simulink model "EulerPIDTunning"  (Simulink 7.6)
settings: Solver=ode3  StartTime=0.0  StopTime=2  FixedStep=Ts  RelTol=1e-3
InitFcn:
  | eval('Config');
  | eval('RobotCtlCfg');
values from neighbouring files (symbols this model uses):
  a2 = 0    [Config.m]    (also in CtrPlatformCfg.m)
  a3 = 0    [Config.m]    (also in CtrPlatformCfg.m)
  a4 = 0    [Config.m]    (also in CtrPlatformCfg.m)
  a5 = 90    [Config.m]    (also in CtrPlatformCfg.m)
  a6 = 0    [Config.m]    (also in CtrPlatformCfg.m)
  freq = tvel/radius    (= 1)    [Config.m]    (also in CtrPlatformCfg.m)
  Gravity = 9.8    [Config.m]    (also in CtrPlatformCfg.m)
  in1 = [5.2954 -0.2565 -0.6366;-0.2565 4.7000 0.2830;-0.6366 0.2829 5.8635]    [Config.m]    (also in CtrPlatformCfg.m; DynEulerTest.m; EfDynCAD.m = [0.54  -0.01 0.23)
  in2 = [5.8840 0.0072 0.0135;0.0072 6.0178 -0.1907;0.0135 -0.1907 0.3374]    [Config.m]    (also in CtrPlatformCfg.m; DynEulerTest.m; EfDynCAD.m = (R_x*R_z)*in2*(R_x*R_z)')
  in3 = [1.8201 -0.2274 -0.3112;-0.2274 2.2537 -0.1441;-0.3112 -0.1441 1.9485]    [Config.m]    (also in CtrPlatformCfg.m; DynEulerTest.m; EfDynCAD.m = (R_x*R_z)*in3*(R_x*R_z)')
  in4 = [0.0607 -0.0922 0;-0.0922 1.4493 0;0 0 1.4620]    [Config.m]    (also in CtrPlatformCfg.m; DynEulerTest.m = [0.0607 -0.0922 0;-0.0922 1.4493 0;0 0,1.4620]; EfDynCAD.m = (R_y*Rz)*in4*(R_y*Rz)')
  in5 = [0.0191 0.0032 0;0.0032 0.0228 0;0 0 0.0291]    [Config.m]    (also in CtrPlatformCfg.m; DynEulerTest.m; EfDynCAD.m = (R_x*R_y)*in5*(R_x*R_y)')
  in6 = [0.0012 0 0;0 0.0007 0;0 0 0.0007]    [Config.m]    (also in CtrPlatformCfg.m; DynEulerTest.m; EfDynCAD.m = (R_y*Rz)*in6*(R_y*Rz)')
  init_Endx = gd_init(1,4)    [Config.m]    (also in CtrPlatformCfg.m)
  init_Endy = gd_init(2,4)    [Config.m]    (also in CtrPlatformCfg.m)
  init_Endz = gd_init(3,4)    [Config.m]    (also in CtrPlatformCfg.m)
  init_Rot = gd_init(1:3,1:3)    [Config.m]    (also in CtrPlatformCfg.m)
  L = [l1 l2 l3 l4 l5 l6 l7 l8 l9]    [Config.m]    (also in CtrPlatformCfg.m)
  ma1 = 170.31    [Config.m]    (also in CtrPlatformCfg.m; DynEulerTest.m; EfDynCAD.m = 77.75)
  ma2 = 63.74    [Config.m]    (also in CtrPlatformCfg.m; DynEulerTest.m; EfDynCAD.m = 32.31)
  ma3 = 98.98    [Config.m]    (also in CtrPlatformCfg.m; DynEulerTest.m; EfDynCAD.m = 18.61)
  ma4 = 24.46    [Config.m]    (also in CtrPlatformCfg.m; DynEulerTest.m; EfDynCAD.m = 15.65)
  ma5 = 5.24    [Config.m]    (also in CtrPlatformCfg.m; DynEulerTest.m; EfDynCAD.m = 3.32)
  ma6 = 0.6    [Config.m]    (also in CtrPlatformCfg.m; DynEulerTest.m; EfDynCAD.m)
  Rad2Line = Gear*EncRes/(2*pi)    [Config.m]    (also in CtrPlatformCfg.m)
  Ts = 1/FrHz    (= 0.00025)    [Config.m]    (also in CtrPlatformCfg.m)
  tvel = 120    [Config.m]    (also in CtrPlatformCfg.m)
undefined symbols (not defined in the file or in its folder): a1, DiscIntNeverNeededParam, PRBSGain, PRBSOffset, PRBSTimeLength, PulseFrq, PulseGain, RobotAxis, SineFrq, SineGain, V2T
libraries: simulink x55, mblibv1 x35, powerlib_extras x7
(part 3 of 3)

== system EulerPIDTunning/Trajectory Generator/Still/Re-group  ==
  JJVVAA : Inport
  Demux2 : Demux  Outputs=18
  Mux{,1..2,4..6} (6 alike) : Mux  Inputs=3
  Mux3 : Mux  Inputs=6
  JVAJVA : Outport
  wires:
  Demux2/18 -> Mux6/3
  Demux2/17 -> Mux5/3
  Demux2/16 -> Mux4/3
  Demux2/15 -> Mux2/3
  Demux2/14 -> Mux1/3
  Demux2/13 -> Mux/3
  Demux2/12 -> Mux6/2
  Demux2/11 -> Mux5/2
  Demux2/10 -> Mux4/2
  Demux2/9 -> Mux2/2
  Demux2/8 -> Mux1/2
  Demux2/7 -> Mux/2
  Demux2/6 -> Mux6/1
  Demux2/5 -> Mux5/1
  Demux2/4 -> Mux4/1
  Demux2/3 -> Mux2/1
  Demux2/2 -> Mux1/1
  Demux2/1 -> Mux/1
  Mux6/1 -> Mux3/6
  Mux5/1 -> Mux3/5
  Mux4/1 -> Mux3/4
  Mux2/1 -> Mux3/3
  Mux1/1 -> Mux3/2
  Mux/1 -> Mux3/1
  Mux3/1 -> JVAJVA/1
  JJVVAA/1 -> Demux2/1

== system EulerPIDTunning/Controller/PID Controller/Controller Axis 1/EncDiff2Vel ==
  Enc : Inport
  Add : Sum  Inputs=+-
  Discrete  2nd-Order Filter : powerlib_extras/Discrete  Control Blocks/Discrete  2nd-Order Filter  DialogController=POWERSYS.PowerSysDialog  SystemSampleTime=-1  FilterType=Lowpass  Fo=1000  Zeta=0.707  Ts=Ts  Initialize=off  Vac_Init=[0.8 -25 60]  Vdc_Init=-0.4  PlotResponse=off  param1=[1 5000 10]
  Integer Delay : simulink/Discrete/Integer Delay  NumDelays=1  InputProcessing=Inherited  vinit=a1/180*pi  samptime=-1
  Vel : Outport
  wires:
  Add/1 -> Discrete  2nd-Order Filter/1
  Discrete  2nd-Order Filter/1 -> Vel/1
  Enc/1 -> Integer Delay/1, Add/1
  Integer Delay/1 -> Add/2

== system EulerPIDTunning/Controller/PID Controller/Controller Axis 1/Error Check and Lock Error ==
  CurrentCheck : Inport
  VelocityCheck : Inport  Port=2
  Abs : Abs
  Abs1 : Abs
  Compare To Constant : simulink/Logic and Bit Operations/Compare To Constant  SystemSampleTime=-1  relop=<=  const=VelErrorCheckLimit  LogicOutDataTypeMode=uint8  ZeroCross=off
  Compare To Constant1 : simulink/Logic and Bit Operations/Compare To Constant  SystemSampleTime=-1  relop=<=  const=VLLimit *1.01  LogicOutDataTypeMode=uint8  ZeroCross=off
  Logical Operator : Logic  Inputs=3  AllPortsSameDT=off  OutDataTypeStr=boolean
  Unit Delay : UnitDelay  X0=1  SampleTime=Ts
  ErrorFlag : Outport
  wires:
  VelocityCheck/1 -> Abs/1
  CurrentCheck/1 -> Abs1/1
  Unit Delay/1 -> Logical Operator/3
  Abs/1 -> Compare To Constant/1
  Abs1/1 -> Compare To Constant1/1
  Compare To Constant1/1 -> Logical Operator/1
  Compare To Constant/1 -> Logical Operator/2
  Logical Operator/1 -> ErrorFlag/1, Unit Delay/1

== system EulerPIDTunning/Controller/PID Controller/Controller Axis 1/PosAdj ==
  Pos : Inport
  Abs : Abs
  Add : Sum  Inputs=+-
  Add1 : Sum  Inputs=+-
  Compare To Constant : simulink/Logic and Bit Operations/Compare To Constant  SystemSampleTime=-1  relop=>=  const=pi/2  LogicOutDataTypeMode=uint8  ZeroCross=off
  Constant : Constant  Value=2*pi  SampleTime=Ts
  Int : DiscreteTransferFcn  Numerator=[1 0]  Denominator=[1 -1]  InitialStates=a1/180*pi  SampleTime=Ts
  Integer Delay : simulink/Discrete/Integer Delay  NumDelays=1  InputProcessing=Inherited  vinit=a1/180*pi  samptime=-1
  Product : Product  RndMeth=Zero
  Product1 : Product  RndMeth=Zero
  Sign : Signum
  PosAdj : Outport
  wires:
  Add1/1 -> Int/1
  Pos/1 -> Add/1, Integer Delay/1
  Int/1 -> PosAdj/1
  Add/1 -> Abs/1, Add1/1, Sign/1
  Integer Delay/1 -> Add/2
  Compare To Constant/1 -> Product/2
  Product/1 -> Add1/2
  Abs/1 -> Compare To Constant/1
  Constant/1 -> Product1/2
  Product1/1 -> Product/1
  Sign/1 -> Product1/1

== system EulerPIDTunning/Controller/PID Controller/Controller Axis 1/controller: PID ==
  Error : Inport
  Add1 : Sum  Inputs=+++
  D : Gain  Gain=Kd
  Diff : simulink/Discrete/Difference  SystemSampleTime=-1  ICPrevInput=0.0  OutMin=[]  OutMax=[]  OutDataType=sfix(16)  OutScaling=2^-10  DoSatur=off
  I : Gain  Gain=Ki
  Int : DiscreteTransferFcn  Numerator=[1 0]  Denominator=[1 -1]  SampleTime=Ts
  Saturation : Saturate  UpperLimit=LimitSet  LowerLimit=-LimitSet  SampleTime=Ts
      settings: AttributesFormatString=%<UpperLimit>\n%<LowerLimit>
  Saturation1 : Saturate  UpperLimit=LimitSet  LowerLimit=-LimitSet  SampleTime=Ts
      settings: AttributesFormatString=%<UpperLimit>\n%<LowerLimit>
  p : Gain  Gain=Kp
  Ctl : Outport
  wires:
  Error/1 -> p/1, I/1, D/1
  p/1 -> Add1/1
  I/1 -> Int/1
  Add1/1 -> Ctl/1
  D/1 -> Diff/1
  Diff/1 -> Saturation1/1
  Int/1 -> Saturation/1
  Saturation/1 -> Add1/2
  Saturation1/1 -> Add1/3

== system EulerPIDTunning/Controller/PID Controller/Controller Axis 1/controller: PID1 ==
  Error : Inport
  Add1 : Sum  Inputs=+++
  D : Gain  Gain=Kd
  Diff : simulink/Discrete/Difference  SystemSampleTime=-1  ICPrevInput=0.0  OutMin=[]  OutMax=[]  OutDataType=sfix(16)  OutScaling=2^-10  DoSatur=off
  I : Gain  Gain=Ki
  Int : DiscreteTransferFcn  Numerator=[1 0]  Denominator=[1 -1]  SampleTime=Ts
  Saturation1 : Saturate  UpperLimit=LimitSet  LowerLimit=-LimitSet  SampleTime=Ts
      settings: AttributesFormatString=%<UpperLimit>\n%<LowerLimit>
  Saturation2 : Saturate  UpperLimit=LimitSet  LowerLimit=-LimitSet  SampleTime=Ts
      settings: AttributesFormatString=%<UpperLimit>\n%<LowerLimit>
  p : Gain  Gain=Kp
  Ctl : Outport
  wires:
  Int/1 -> Saturation2/1
  Diff/1 -> Saturation1/1
  D/1 -> Diff/1
  Add1/1 -> Ctl/1
  I/1 -> Int/1
  p/1 -> Add1/1
  Error/1 -> D/1, I/1, p/1
  Saturation2/1 -> Add1/2
  Saturation1/1 -> Add1/3

== system EulerPIDTunning/Controller/PID Controller/Controller Axis 2/EncDiff2Vel ==
  Enc : Inport
  Add : Sum  Inputs=+-
  Discrete  2nd-Order Filter : powerlib_extras/Discrete  Control Blocks/Discrete  2nd-Order Filter  DialogController=POWERSYS.PowerSysDialog  SystemSampleTime=-1  FilterType=Lowpass  Fo=1000  Zeta=0.707  Ts=Ts  Initialize=off  Vac_Init=[0.8 -25 60]  Vdc_Init=-0.4  PlotResponse=off  param1=[1 5000 10]
  Integer Delay : simulink/Discrete/Integer Delay  NumDelays=1  InputProcessing=Inherited  vinit=a2/180*pi  samptime=-1
  Vel : Outport
  wires:
  Integer Delay/1 -> Add/2
  Enc/1 -> Add/1, Integer Delay/1
  Discrete  2nd-Order Filter/1 -> Vel/1
  Add/1 -> Discrete  2nd-Order Filter/1

== system EulerPIDTunning/Controller/PID Controller/Controller Axis 2/Error Check and Lock Error ==
  CurrentCheck : Inport
  VelocityCheck : Inport  Port=2
  Abs : Abs
  Abs1 : Abs
  Compare To Constant : simulink/Logic and Bit Operations/Compare To Constant  SystemSampleTime=-1  relop=<=  const=VelErrorCheckLimit  LogicOutDataTypeMode=uint8  ZeroCross=off
  Compare To Constant1 : simulink/Logic and Bit Operations/Compare To Constant  SystemSampleTime=-1  relop=<=  const=VLLimit *1.01  LogicOutDataTypeMode=uint8  ZeroCross=off
  Logical Operator : Logic  Inputs=3  AllPortsSameDT=off  OutDataTypeStr=boolean
  Unit Delay : UnitDelay  X0=1  SampleTime=Ts
  ErrorFlag : Outport
  wires:
  Logical Operator/1 -> Unit Delay/1, ErrorFlag/1
  Compare To Constant/1 -> Logical Operator/2
  Compare To Constant1/1 -> Logical Operator/1
  Abs1/1 -> Compare To Constant1/1
  Abs/1 -> Compare To Constant/1
  Unit Delay/1 -> Logical Operator/3
  CurrentCheck/1 -> Abs1/1
  VelocityCheck/1 -> Abs/1

== system EulerPIDTunning/Controller/PID Controller/Controller Axis 2/PosAdj ==
  Pos : Inport
  Abs : Abs
  Add : Sum  Inputs=+-
  Add1 : Sum  Inputs=+-
  Compare To Constant : simulink/Logic and Bit Operations/Compare To Constant  SystemSampleTime=-1  relop=>=  const=pi/2  LogicOutDataTypeMode=uint8  ZeroCross=off
  Constant : Constant  Value=2*pi  SampleTime=Ts
  Int : DiscreteTransferFcn  Numerator=[1 0]  Denominator=[1 -1]  InitialStates=a2/180*pi  SampleTime=Ts
  Integer Delay : simulink/Discrete/Integer Delay  NumDelays=1  InputProcessing=Inherited  vinit=a2/180*pi  samptime=-1
  Product : Product  RndMeth=Zero
  Product1 : Product  RndMeth=Zero
  Sign : Signum
  PosAdj : Outport
  wires:
  Add1/1 -> Int/1
  Pos/1 -> Add/1, Integer Delay/1
  Int/1 -> PosAdj/1
  Add/1 -> Abs/1, Add1/1, Sign/1
  Integer Delay/1 -> Add/2
  Compare To Constant/1 -> Product/2
  Product/1 -> Add1/2
  Abs/1 -> Compare To Constant/1
  Constant/1 -> Product1/2
  Product1/1 -> Product/1
  Sign/1 -> Product1/1

== system EulerPIDTunning/Controller/PID Controller/Controller Axis 2/controller: PID ==
  Error : Inport
  Add1 : Sum  Inputs=+++
  D : Gain  Gain=Kd
  Diff : simulink/Discrete/Difference  SystemSampleTime=-1  ICPrevInput=0.0  OutMin=[]  OutMax=[]  OutDataType=sfix(16)  OutScaling=2^-10  DoSatur=off
  I : Gain  Gain=Ki
  Int : DiscreteTransferFcn  Numerator=[1 0]  Denominator=[1 -1]  SampleTime=Ts
  Saturation : Saturate  UpperLimit=LimitSet  LowerLimit=-LimitSet  SampleTime=Ts
      settings: AttributesFormatString=%<UpperLimit>\n%<LowerLimit>
  Saturation1 : Saturate  UpperLimit=LimitSet  LowerLimit=-LimitSet  SampleTime=Ts
      settings: AttributesFormatString=%<UpperLimit>\n%<LowerLimit>
  p : Gain  Gain=Kp
  Ctl : Outport
  wires:
  Saturation1/1 -> Add1/3
  Saturation/1 -> Add1/2
  Int/1 -> Saturation/1
  Diff/1 -> Saturation1/1
  D/1 -> Diff/1
  Add1/1 -> Ctl/1
  I/1 -> Int/1
  p/1 -> Add1/1
  Error/1 -> D/1, I/1, p/1

== system EulerPIDTunning/Controller/PID Controller/Controller Axis 2/controller: PID1 ==
  Error : Inport
  Add1 : Sum  Inputs=+++
  D : Gain  Gain=Kd
  Diff : simulink/Discrete/Difference  SystemSampleTime=-1  ICPrevInput=0.0  OutMin=[]  OutMax=[]  OutDataType=sfix(16)  OutScaling=2^-10  DoSatur=off
  I : Gain  Gain=Ki
  Int : DiscreteTransferFcn  Numerator=[1 0]  Denominator=[1 -1]  SampleTime=Ts
  Saturation1 : Saturate  UpperLimit=LimitSet  LowerLimit=-LimitSet  SampleTime=Ts
      settings: AttributesFormatString=%<UpperLimit>\n%<LowerLimit>
  Saturation2 : Saturate  UpperLimit=LimitSet  LowerLimit=-LimitSet  SampleTime=Ts
      settings: AttributesFormatString=%<UpperLimit>\n%<LowerLimit>
  p : Gain  Gain=Kp
  Ctl : Outport
  wires:
  Saturation1/1 -> Add1/3
  Saturation2/1 -> Add1/2
  Error/1 -> p/1, I/1, D/1
  p/1 -> Add1/1
  I/1 -> Int/1
  Add1/1 -> Ctl/1
  D/1 -> Diff/1
  Diff/1 -> Saturation1/1
  Int/1 -> Saturation2/1

== system EulerPIDTunning/Controller/PID Controller/Controller Axis 3/EncDiff2Vel ==
  Enc : Inport
  Add : Sum  Inputs=+-
  Discrete  2nd-Order Filter : powerlib_extras/Discrete  Control Blocks/Discrete  2nd-Order Filter  DialogController=POWERSYS.PowerSysDialog  SystemSampleTime=-1  FilterType=Lowpass  Fo=1000  Zeta=0.707  Ts=Ts  Initialize=off  Vac_Init=[0.8 -25 60]  Vdc_Init=-0.4  PlotResponse=off  param1=[1 5000 10]
  Integer Delay : simulink/Discrete/Integer Delay  NumDelays=1  InputProcessing=Inherited  vinit=a3/180*pi  samptime=-1
  Vel : Outport
  wires:
  Add/1 -> Discrete  2nd-Order Filter/1
  Discrete  2nd-Order Filter/1 -> Vel/1
  Enc/1 -> Integer Delay/1, Add/1
  Integer Delay/1 -> Add/2

== system EulerPIDTunning/Controller/PID Controller/Controller Axis 3/Error Check and Lock Error ==
  CurrentCheck : Inport
  VelocityCheck : Inport  Port=2
  Abs : Abs
  Abs1 : Abs
  Compare To Constant : simulink/Logic and Bit Operations/Compare To Constant  SystemSampleTime=-1  relop=<=  const=VelErrorCheckLimit  LogicOutDataTypeMode=uint8  ZeroCross=off
  Compare To Constant1 : simulink/Logic and Bit Operations/Compare To Constant  SystemSampleTime=-1  relop=<=  const=VLLimit *1.01  LogicOutDataTypeMode=uint8  ZeroCross=off
  Logical Operator : Logic  Inputs=3  AllPortsSameDT=off  OutDataTypeStr=boolean
  Unit Delay : UnitDelay  X0=1  SampleTime=Ts
  ErrorFlag : Outport
  wires:
  VelocityCheck/1 -> Abs/1
  CurrentCheck/1 -> Abs1/1
  Unit Delay/1 -> Logical Operator/3
  Abs/1 -> Compare To Constant/1
  Abs1/1 -> Compare To Constant1/1
  Compare To Constant1/1 -> Logical Operator/1
  Compare To Constant/1 -> Logical Operator/2
  Logical Operator/1 -> ErrorFlag/1, Unit Delay/1

== system EulerPIDTunning/Controller/PID Controller/Controller Axis 3/PosAdj ==
  Pos : Inport
  Abs : Abs
  Add : Sum  Inputs=+-
  Add1 : Sum  Inputs=+-
  Compare To Constant : simulink/Logic and Bit Operations/Compare To Constant  SystemSampleTime=-1  relop=>=  const=pi/2  LogicOutDataTypeMode=uint8  ZeroCross=off
  Constant : Constant  Value=2*pi  SampleTime=Ts
  Int : DiscreteTransferFcn  Numerator=[1 0]  Denominator=[1 -1]  InitialStates=a3/180*pi  SampleTime=Ts
  Integer Delay : simulink/Discrete/Integer Delay  NumDelays=1  InputProcessing=Inherited  vinit=a3/180*pi  samptime=-1
  Product : Product  RndMeth=Zero
  Product1 : Product  RndMeth=Zero
  Sign : Signum
  PosAdj : Outport
  wires:
  Add1/1 -> Int/1
  Pos/1 -> Add/1, Integer Delay/1
  Int/1 -> PosAdj/1
  Add/1 -> Abs/1, Add1/1, Sign/1
  Integer Delay/1 -> Add/2
  Compare To Constant/1 -> Product/2
  Product/1 -> Add1/2
  Abs/1 -> Compare To Constant/1
  Constant/1 -> Product1/2
  Product1/1 -> Product/1
  Sign/1 -> Product1/1

== system EulerPIDTunning/Controller/PID Controller/Controller Axis 3/controller: PID ==
  Error : Inport
  Add1 : Sum  Inputs=+++
  D : Gain  Gain=Kd
  Diff : simulink/Discrete/Difference  SystemSampleTime=-1  ICPrevInput=0.0  OutMin=[]  OutMax=[]  OutDataType=sfix(16)  OutScaling=2^-10  DoSatur=off
  I : Gain  Gain=Ki
  Int : DiscreteTransferFcn  Numerator=[1 0]  Denominator=[1 -1]  SampleTime=Ts
  Saturation : Saturate  UpperLimit=LimitSet  LowerLimit=-LimitSet  SampleTime=Ts
      settings: AttributesFormatString=%<UpperLimit>\n%<LowerLimit>
  Saturation1 : Saturate  UpperLimit=LimitSet  LowerLimit=-LimitSet  SampleTime=Ts
      settings: AttributesFormatString=%<UpperLimit>\n%<LowerLimit>
  p : Gain  Gain=Kp
  Ctl : Outport
  wires:
  Error/1 -> p/1, I/1, D/1
  p/1 -> Add1/1
  I/1 -> Int/1
  Add1/1 -> Ctl/1
  D/1 -> Diff/1
  Diff/1 -> Saturation1/1
  Int/1 -> Saturation/1
  Saturation/1 -> Add1/2
  Saturation1/1 -> Add1/3

== system EulerPIDTunning/Controller/PID Controller/Controller Axis 3/controller: PID1 ==
  Error : Inport
  Add1 : Sum  Inputs=+++
  D : Gain  Gain=Kd
  Diff : simulink/Discrete/Difference  SystemSampleTime=-1  ICPrevInput=0.0  OutMin=[]  OutMax=[]  OutDataType=sfix(16)  OutScaling=2^-10  DoSatur=off
  I : Gain  Gain=Ki
  Int : DiscreteTransferFcn  Numerator=[1 0]  Denominator=[1 -1]  SampleTime=Ts
  Saturation1 : Saturate  UpperLimit=LimitSet  LowerLimit=-LimitSet  SampleTime=Ts
      settings: AttributesFormatString=%<UpperLimit>\n%<LowerLimit>
  Saturation2 : Saturate  UpperLimit=LimitSet  LowerLimit=-LimitSet  SampleTime=Ts
      settings: AttributesFormatString=%<UpperLimit>\n%<LowerLimit>
  p : Gain  Gain=Kp
  Ctl : Outport
  wires:
  Int/1 -> Saturation2/1
  Diff/1 -> Saturation1/1
  D/1 -> Diff/1
  Add1/1 -> Ctl/1
  I/1 -> Int/1
  p/1 -> Add1/1
  Error/1 -> D/1, I/1, p/1
  Saturation2/1 -> Add1/2
  Saturation1/1 -> Add1/3

== system EulerPIDTunning/Controller/PID Controller/Controller Axis 4/EncDiff2Vel ==
  Enc : Inport
  Add : Sum  Inputs=+-
  Discrete  2nd-Order Filter : powerlib_extras/Discrete  Control Blocks/Discrete  2nd-Order Filter  DialogController=POWERSYS.PowerSysDialog  SystemSampleTime=-1  FilterType=Lowpass  Fo=1000  Zeta=0.707  Ts=Ts  Initialize=off  Vac_Init=[0.8 -25 60]  Vdc_Init=-0.4  PlotResponse=off  param1=[1 5000 10]
  Integer Delay : simulink/Discrete/Integer Delay  NumDelays=1  InputProcessing=Inherited  vinit=a4/180*pi  samptime=-1
  Vel : Outport
  wires:
  Integer Delay/1 -> Add/2
  Enc/1 -> Add/1, Integer Delay/1
  Discrete  2nd-Order Filter/1 -> Vel/1
  Add/1 -> Discrete  2nd-Order Filter/1

== system EulerPIDTunning/Controller/PID Controller/Controller Axis 4/Error Check and Lock Error ==
  CurrentCheck : Inport
  VelocityCheck : Inport  Port=2
  Abs : Abs
  Abs1 : Abs
  Compare To Constant : simulink/Logic and Bit Operations/Compare To Constant  SystemSampleTime=-1  relop=<=  const=VelErrorCheckLimit  LogicOutDataTypeMode=uint8  ZeroCross=off
  Compare To Constant1 : simulink/Logic and Bit Operations/Compare To Constant  SystemSampleTime=-1  relop=<=  const=VLLimit *1.01  LogicOutDataTypeMode=uint8  ZeroCross=off
  Logical Operator : Logic  Inputs=3  AllPortsSameDT=off  OutDataTypeStr=boolean
  Unit Delay : UnitDelay  X0=1  SampleTime=Ts
  ErrorFlag : Outport
  wires:
  Logical Operator/1 -> Unit Delay/1, ErrorFlag/1
  Compare To Constant/1 -> Logical Operator/2
  Compare To Constant1/1 -> Logical Operator/1
  Abs1/1 -> Compare To Constant1/1
  Abs/1 -> Compare To Constant/1
  Unit Delay/1 -> Logical Operator/3
  CurrentCheck/1 -> Abs1/1
  VelocityCheck/1 -> Abs/1

== system EulerPIDTunning/Controller/PID Controller/Controller Axis 4/PosAdj ==
  Pos : Inport
  Abs : Abs
  Add : Sum  Inputs=+-
  Add1 : Sum  Inputs=+-
  Compare To Constant : simulink/Logic and Bit Operations/Compare To Constant  SystemSampleTime=-1  relop=>=  const=pi/2  LogicOutDataTypeMode=uint8  ZeroCross=off
  Constant : Constant  Value=2*pi  SampleTime=Ts
  Int : DiscreteTransferFcn  Numerator=[1 0]  Denominator=[1 -1]  SampleTime=Ts
  Integer Delay : simulink/Discrete/Integer Delay  NumDelays=1  InputProcessing=Inherited  vinit=a4/180*pi  samptime=-1
  Product : Product  RndMeth=Zero
  Product1 : Product  RndMeth=Zero
  Sign : Signum
  PosAdj : Outport
  wires:
  Add1/1 -> Int/1
  Pos/1 -> Add/1, Integer Delay/1
  Int/1 -> PosAdj/1
  Add/1 -> Abs/1, Add1/1, Sign/1
  Integer Delay/1 -> Add/2
  Compare To Constant/1 -> Product/2
  Product/1 -> Add1/2
  Abs/1 -> Compare To Constant/1
  Constant/1 -> Product1/2
  Product1/1 -> Product/1
  Sign/1 -> Product1/1

== system EulerPIDTunning/Controller/PID Controller/Controller Axis 4/controller: PID ==
  Error : Inport
  Add1 : Sum  Inputs=+++
  D : Gain  Gain=Kd
  Diff : simulink/Discrete/Difference  SystemSampleTime=-1  ICPrevInput=0.0  OutMin=[]  OutMax=[]  OutDataType=sfix(16)  OutScaling=2^-10  DoSatur=off
  I : Gain  Gain=Ki
  Int : DiscreteTransferFcn  Numerator=[1 0]  Denominator=[1 -1]  SampleTime=Ts
  Saturation : Saturate  UpperLimit=LimitSet  LowerLimit=-LimitSet  SampleTime=Ts
      settings: AttributesFormatString=%<UpperLimit>\n%<LowerLimit>
  Saturation1 : Saturate  UpperLimit=LimitSet  LowerLimit=-LimitSet  SampleTime=Ts
      settings: AttributesFormatString=%<UpperLimit>\n%<LowerLimit>
  p : Gain  Gain=Kp
  Ctl : Outport
  wires:
  Saturation1/1 -> Add1/3
  Saturation/1 -> Add1/2
  Int/1 -> Saturation/1
  Diff/1 -> Saturation1/1
  D/1 -> Diff/1
  Add1/1 -> Ctl/1
  I/1 -> Int/1
  p/1 -> Add1/1
  Error/1 -> D/1, I/1, p/1

== system EulerPIDTunning/Controller/PID Controller/Controller Axis 4/controller: PID1 ==
  Error : Inport
  Add1 : Sum  Inputs=+++
  D : Gain  Gain=Kd
  Diff : simulink/Discrete/Difference  SystemSampleTime=-1  ICPrevInput=0.0  OutMin=[]  OutMax=[]  OutDataType=sfix(16)  OutScaling=2^-10  DoSatur=off
  I : Gain  Gain=Ki
  Int : DiscreteTransferFcn  Numerator=[1 0]  Denominator=[1 -1]  SampleTime=Ts
  Saturation1 : Saturate  UpperLimit=LimitSet  LowerLimit=-LimitSet  SampleTime=Ts
      settings: AttributesFormatString=%<UpperLimit>\n%<LowerLimit>
  Saturation2 : Saturate  UpperLimit=LimitSet  LowerLimit=-LimitSet  SampleTime=Ts
      settings: AttributesFormatString=%<UpperLimit>\n%<LowerLimit>
  p : Gain  Gain=Kp
  Ctl : Outport
  wires:
  Saturation1/1 -> Add1/3
  Saturation2/1 -> Add1/2
  Error/1 -> p/1, I/1, D/1
  p/1 -> Add1/1
  I/1 -> Int/1
  Add1/1 -> Ctl/1
  D/1 -> Diff/1
  Diff/1 -> Saturation1/1
  Int/1 -> Saturation2/1

== system EulerPIDTunning/Controller/PID Controller/Controller Axis 5/EncDiff2Vel ==
  Enc : Inport
  Add : Sum  Inputs=+-
  Discrete  2nd-Order Filter : powerlib_extras/Discrete  Control Blocks/Discrete  2nd-Order Filter  DialogController=POWERSYS.PowerSysDialog  SystemSampleTime=-1  FilterType=Lowpass  Fo=1000  Zeta=0.707  Ts=Ts  Initialize=off  Vac_Init=[0.8 -25 60]  Vdc_Init=-0.4  PlotResponse=off  param1=[1 5000 10]
  Integer Delay : simulink/Discrete/Integer Delay  NumDelays=1  InputProcessing=Inherited  vinit=a5/180*pi  samptime=-1
  Vel : Outport
  wires:
  Add/1 -> Discrete  2nd-Order Filter/1
  Discrete  2nd-Order Filter/1 -> Vel/1
  Enc/1 -> Integer Delay/1, Add/1
  Integer Delay/1 -> Add/2

== system EulerPIDTunning/Controller/PID Controller/Controller Axis 5/Error Check and Lock Error ==
  CurrentCheck : Inport
  VelocityCheck : Inport  Port=2
  Abs : Abs
  Abs1 : Abs
  Compare To Constant : simulink/Logic and Bit Operations/Compare To Constant  SystemSampleTime=-1  relop=<=  const=VelErrorCheckLimit  LogicOutDataTypeMode=uint8  ZeroCross=off
  Compare To Constant1 : simulink/Logic and Bit Operations/Compare To Constant  SystemSampleTime=-1  relop=<=  const=VLLimit *1.01  LogicOutDataTypeMode=uint8  ZeroCross=off
  Logical Operator : Logic  Inputs=3  AllPortsSameDT=off  OutDataTypeStr=boolean
  Unit Delay : UnitDelay  X0=1  SampleTime=Ts
  ErrorFlag : Outport
  wires:
  VelocityCheck/1 -> Abs/1
  CurrentCheck/1 -> Abs1/1
  Unit Delay/1 -> Logical Operator/3
  Abs/1 -> Compare To Constant/1
  Abs1/1 -> Compare To Constant1/1
  Compare To Constant1/1 -> Logical Operator/1
  Compare To Constant/1 -> Logical Operator/2
  Logical Operator/1 -> ErrorFlag/1, Unit Delay/1

== system EulerPIDTunning/Controller/PID Controller/Controller Axis 5/PosAdj ==
  Pos : Inport
  Abs : Abs
  Add : Sum  Inputs=+-
  Add1 : Sum  Inputs=+-
  Compare To Constant : simulink/Logic and Bit Operations/Compare To Constant  SystemSampleTime=-1  relop=>=  const=pi/2  LogicOutDataTypeMode=uint8  ZeroCross=off
  Constant : Constant  Value=2*pi  SampleTime=Ts
  Int : DiscreteTransferFcn  Numerator=[1 0]  Denominator=[1 -1]  InitialStates=a5/180*pi  SampleTime=Ts
  Integer Delay : simulink/Discrete/Integer Delay  NumDelays=1  InputProcessing=Inherited  vinit=a5/180*pi  samptime=Ts
  Product : Product  RndMeth=Zero
  Product1 : Product  RndMeth=Zero
  Sign : Signum
  PosAdj : Outport
  wires:
  Add1/1 -> Int/1
  Pos/1 -> Add/1, Integer Delay/1
  Int/1 -> PosAdj/1
  Add/1 -> Abs/1, Add1/1, Sign/1
  Integer Delay/1 -> Add/2
  Compare To Constant/1 -> Product/2
  Product/1 -> Add1/2
  Abs/1 -> Compare To Constant/1
  Constant/1 -> Product1/2
  Product1/1 -> Product/1
  Sign/1 -> Product1/1

== system EulerPIDTunning/Controller/PID Controller/Controller Axis 5/controller: PID ==
  Error : Inport
  Add1 : Sum  Inputs=+++
  D : Gain  Gain=Kd
  Diff : simulink/Discrete/Difference  SystemSampleTime=-1  ICPrevInput=0.0  OutMin=[]  OutMax=[]  OutDataType=sfix(16)  OutScaling=2^-10  DoSatur=off
  I : Gain  Gain=Ki
  Int : DiscreteTransferFcn  Numerator=[1 0]  Denominator=[1 -1]  SampleTime=Ts
  Saturation : Saturate  UpperLimit=LimitSet  LowerLimit=-LimitSet  SampleTime=Ts
      settings: AttributesFormatString=%<UpperLimit>\n%<LowerLimit>
  Saturation1 : Saturate  UpperLimit=LimitSet  LowerLimit=-LimitSet  SampleTime=Ts
      settings: AttributesFormatString=%<UpperLimit>\n%<LowerLimit>
  p : Gain  Gain=Kp
  Ctl : Outport
  wires:
  Error/1 -> p/1, I/1, D/1
  p/1 -> Add1/1
  I/1 -> Int/1
  Add1/1 -> Ctl/1
  D/1 -> Diff/1
  Diff/1 -> Saturation1/1
  Int/1 -> Saturation/1
  Saturation/1 -> Add1/2
  Saturation1/1 -> Add1/3

== system EulerPIDTunning/Controller/PID Controller/Controller Axis 5/controller: PID1 ==
  Error : Inport
  Add1 : Sum  Inputs=+++
  D : Gain  Gain=Kd
  Diff : simulink/Discrete/Difference  SystemSampleTime=-1  ICPrevInput=0.0  OutMin=[]  OutMax=[]  OutDataType=sfix(16)  OutScaling=2^-10  DoSatur=off
  I : Gain  Gain=Ki
  Int : DiscreteTransferFcn  Numerator=[1 0]  Denominator=[1 -1]  SampleTime=Ts
  Saturation1 : Saturate  UpperLimit=LimitSet  LowerLimit=-LimitSet  SampleTime=Ts
      settings: AttributesFormatString=%<UpperLimit>\n%<LowerLimit>
  Saturation2 : Saturate  UpperLimit=LimitSet  LowerLimit=-LimitSet  SampleTime=Ts
      settings: AttributesFormatString=%<UpperLimit>\n%<LowerLimit>
  p : Gain  Gain=Kp
  Ctl : Outport
  wires:
  Int/1 -> Saturation2/1
  Diff/1 -> Saturation1/1
  D/1 -> Diff/1
  Add1/1 -> Ctl/1
  I/1 -> Int/1
  p/1 -> Add1/1
  Error/1 -> D/1, I/1, p/1
  Saturation2/1 -> Add1/2
  Saturation1/1 -> Add1/3

== system EulerPIDTunning/Controller/PID Controller/Controller Axis 6/EncDiff2Vel ==
  Enc : Inport
  Add : Sum  Inputs=+-
  Discrete  2nd-Order Filter : powerlib_extras/Discrete  Control Blocks/Discrete  2nd-Order Filter  DialogController=POWERSYS.PowerSysDialog  SystemSampleTime=-1  FilterType=Lowpass  Fo=1000  Zeta=0.707  Ts=Ts  Initialize=off  Vac_Init=[0.8 -25 60]  Vdc_Init=-0.4  PlotResponse=off  param1=[1 5000 10]
  Integer Delay : simulink/Discrete/Integer Delay  NumDelays=1  InputProcessing=Inherited  vinit=a6/180*pi  samptime=-1
  Vel : Outport
  wires:
  Integer Delay/1 -> Add/2
  Enc/1 -> Add/1, Integer Delay/1
  Discrete  2nd-Order Filter/1 -> Vel/1
  Add/1 -> Discrete  2nd-Order Filter/1

== system EulerPIDTunning/Controller/PID Controller/Controller Axis 6/Error Check and Lock Error ==
  CurrentCheck : Inport
  VelocityCheck : Inport  Port=2
  Abs : Abs
  Abs1 : Abs
  Compare To Constant : simulink/Logic and Bit Operations/Compare To Constant  SystemSampleTime=-1  relop=<=  const=VelErrorCheckLimit  LogicOutDataTypeMode=uint8  ZeroCross=off
  Compare To Constant1 : simulink/Logic and Bit Operations/Compare To Constant  SystemSampleTime=-1  relop=<=  const=VLLimit *1.01  LogicOutDataTypeMode=uint8  ZeroCross=off
  Logical Operator : Logic  Inputs=3  AllPortsSameDT=off  OutDataTypeStr=boolean
  Unit Delay : UnitDelay  X0=1  SampleTime=Ts
  ErrorFlag : Outport
  wires:
  Logical Operator/1 -> Unit Delay/1, ErrorFlag/1
  Compare To Constant/1 -> Logical Operator/2
  Compare To Constant1/1 -> Logical Operator/1
  Abs1/1 -> Compare To Constant1/1
  Abs/1 -> Compare To Constant/1
  Unit Delay/1 -> Logical Operator/3
  CurrentCheck/1 -> Abs1/1
  VelocityCheck/1 -> Abs/1

== system EulerPIDTunning/Controller/PID Controller/Controller Axis 6/PosAdj ==
  Pos : Inport
  Abs : Abs
  Add : Sum  Inputs=+-
  Add1 : Sum  Inputs=+-
  Compare To Constant : simulink/Logic and Bit Operations/Compare To Constant  SystemSampleTime=-1  relop=>=  const=pi/2  LogicOutDataTypeMode=uint8  ZeroCross=off
  Constant : Constant  Value=2*pi  SampleTime=Ts
  Int : DiscreteTransferFcn  Numerator=[1 0]  Denominator=[1 -1]  InitialStates=a6/180*pi  SampleTime=Ts
  Integer Delay : simulink/Discrete/Integer Delay  NumDelays=1  InputProcessing=Inherited  vinit=a6/180*pi  samptime=-1
  Product : Product  RndMeth=Zero
  Product1 : Product  RndMeth=Zero
  Sign : Signum
  PosAdj : Outport
  wires:
  Add1/1 -> Int/1
  Pos/1 -> Add/1, Integer Delay/1
  Int/1 -> PosAdj/1
  Add/1 -> Abs/1, Add1/1, Sign/1
  Integer Delay/1 -> Add/2
  Compare To Constant/1 -> Product/2
  Product/1 -> Add1/2
  Abs/1 -> Compare To Constant/1
  Constant/1 -> Product1/2
  Product1/1 -> Product/1
  Sign/1 -> Product1/1

== system EulerPIDTunning/Controller/PID Controller/Controller Axis 6/controller: PID ==
  Error : Inport
  Add1 : Sum  Inputs=+++
  D : Gain  Gain=Kd
  Diff : simulink/Discrete/Difference  SystemSampleTime=-1  ICPrevInput=0.0  OutMin=[]  OutMax=[]  OutDataType=sfix(16)  OutScaling=2^-10  DoSatur=off
  I : Gain  Gain=Ki
  Int : DiscreteTransferFcn  Numerator=[1 0]  Denominator=[1 -1]  SampleTime=Ts
  Saturation : Saturate  UpperLimit=LimitSet  LowerLimit=-LimitSet  SampleTime=Ts
      settings: AttributesFormatString=%<UpperLimit>\n%<LowerLimit>
  Saturation1 : Saturate  UpperLimit=LimitSet  LowerLimit=-LimitSet  SampleTime=Ts
      settings: AttributesFormatString=%<UpperLimit>\n%<LowerLimit>
  p : Gain  Gain=Kp
  Ctl : Outport
  wires:
  Saturation1/1 -> Add1/3
  Saturation/1 -> Add1/2
  Int/1 -> Saturation/1
  Diff/1 -> Saturation1/1
  D/1 -> Diff/1
  Add1/1 -> Ctl/1
  I/1 -> Int/1
  p/1 -> Add1/1
  Error/1 -> D/1, I/1, p/1

== system EulerPIDTunning/Controller/PID Controller/Controller Axis 6/controller: PID1 ==
  Error : Inport
  Add1 : Sum  Inputs=+++
  D : Gain  Gain=Kd
  Diff : simulink/Discrete/Difference  SystemSampleTime=-1  ICPrevInput=0.0  OutMin=[]  OutMax=[]  OutDataType=sfix(16)  OutScaling=2^-10  DoSatur=off
  I : Gain  Gain=Ki
  Int : DiscreteTransferFcn  Numerator=[1 0]  Denominator=[1 -1]  SampleTime=Ts
  Saturation1 : Saturate  UpperLimit=LimitSet  LowerLimit=-LimitSet  SampleTime=Ts
      settings: AttributesFormatString=%<UpperLimit>\n%<LowerLimit>
  Saturation2 : Saturate  UpperLimit=LimitSet  LowerLimit=-LimitSet  SampleTime=Ts
      settings: AttributesFormatString=%<UpperLimit>\n%<LowerLimit>
  p : Gain  Gain=Kp
  Ctl : Outport
  wires:
  Saturation1/1 -> Add1/3
  Saturation2/1 -> Add1/2
  Error/1 -> p/1, I/1, D/1
  p/1 -> Add1/1
  I/1 -> Int/1
  Add1/1 -> Ctl/1
  D/1 -> Diff/1
  Diff/1 -> Saturation1/1
  Int/1 -> Saturation2/1

== system EulerPIDTunning/Controller/PID Controller/Source Model/EncDiff2Vel ==
  Enc : Inport
  Add : Sum  Inputs=+-
  Discrete  2nd-Order Filter : powerlib_extras/Discrete  Control Blocks/Discrete  2nd-Order Filter  DialogController=POWERSYS.PowerSysDialog  SystemSampleTime=-1  FilterType=Lowpass  Fo=1000  Zeta=0.707  Ts=Ts  Initialize=off  Vac_Init=[0.8 -25 60]  Vdc_Init=-0.4  PlotResponse=off  param1=[1 5000 10]
  Integer Delay : simulink/Discrete/Integer Delay  NumDelays=1  InputProcessing=Inherited  vinit=0.0  samptime=-1
  Vel : Outport
  wires:
  Integer Delay/1 -> Add/2
  Enc/1 -> Add/1, Integer Delay/1
  Discrete  2nd-Order Filter/1 -> Vel/1
  Add/1 -> Discrete  2nd-Order Filter/1

== system EulerPIDTunning/Controller/PID Controller/Source Model/source: PRBS ==
  Enable : EnablePort  StatesWhenEnabling=reset
  Add : Sum
  Gain1 : Gain  Gain=Ts
  Lookup Table : Lookup  InputValues=(0:TL/Ts)*Ts;  Table=[prbs_u; 0];  LookUpMeth=Interpolation-Use End Values  SampleTime=Ts
  PRBSGain : Gain  Gain=CurrentValue  SampleTime=Ts
  Ts : Constant  SampleTime=Ts
  Unit Delay : UnitDelay  SampleTime=Ts
  PRBS* : Outport  OutputWhenDisabled=reset  InitialOutput=0
  wires:
  Lookup Table/1 -> PRBSGain/1
  PRBSGain/1 -> PRBS*/1
  Add/1 -> Unit Delay/1, Gain1/1
  Ts/1 -> Add/2
  Unit Delay/1 -> Add/1
  Gain1/1 -> Lookup Table/1

== system EulerPIDTunning/Controller/PID Controller/Source Model/source: Pulse ==
  Enable : EnablePort  StatesWhenEnabling=reset
  Add : Sum
  Gain1 : Gain  Gain=Ts
  PulseGain : Gain  Gain=VelGain
  Sign : Signum
  Sine Wave : Sin  TimeSource=Use external signal  Frequency=Frq*2*pi  SampleTime=31.25e-6
  Ts : Constant  SampleTime=Ts
  Unit Delay : UnitDelay  SampleTime=Ts
  Vel1 : Scope
      settings: TimeRange=4.5  YMin=0.15  YMax=1  SaveName=ScopeData10
  Pulse : Outport  OutputWhenDisabled=reset  InitialOutput=0
  wires:
  Sine Wave/1 -> Sign/1, Vel1/1
  Sign/1 -> PulseGain/1
  PulseGain/1 -> Pulse/1
  Add/1 -> Unit Delay/1, Gain1/1
  Ts/1 -> Add/2
  Unit Delay/1 -> Add/1
  Gain1/1 -> Sine Wave/1

== system EulerPIDTunning/Controller/PID Controller/Source Model/source: SineSwp ==
  Enable : EnablePort  StatesWhenEnabling=reset
  AmpG : Subsystem
  Constant : Constant  Value=2*pi  SampleTime=Ts
  DelayCmp : Subsystem
  Product : Product  Inputs=3  RndMeth=Zero
  Product1 : Product  RndMeth=Zero
  Product2 : Product  RndMeth=Zero
  Product3 : Product  RndMeth=Zero
  Scope1 : Scope
      settings: TimeRange=0.05  SaveName=ScopeData3
  Scope4 : Scope
      settings: TimeRange=0.05  SaveName=ScopeData7
  SignalGen : Stateflow chart  TreatAsAtomicUnit=on
  Timer : Subsystem
  Trigonometric Function : Trigonometry  SampleTime=Ts
  Unit Delay1 : UnitDelay  X0=1  SampleTime=Ts
  Unit Delay2 : UnitDelay  SampleTime=Ts
  Unit Delay3 : UnitDelay  X0=1  SampleTime=Ts
  Unit Delay4 : UnitDelay  X0=0.01  SampleTime=Ts
  SineOut : Outport  OutputWhenDisabled=reset  InitialOutput=0
  wires:
  Timer/1(Time) -> Product/1, SignalGen/1(mytime)
  Constant/1 -> Product/2
  SignalGen/1(Frq) -> Product/3, Scope1/1, Unit Delay4/1
  Product/1 -> Trigonometric Function/1
  Product1/1 -> SineOut/1, Scope4/1
  Trigonometric Function/1 -> Product1/1
  AmpG/1(TrueAmp) -> Product1/2, Unit Delay2/1
  Unit Delay2/1 -> SignalGen/2(TureAmp)
  SignalGen/4(CounterOut) -> Unit Delay3/1
  Unit Delay3/1 -> SignalGen/3(CounterIn)
  SignalGen/3(PeriodFlag) -> Unit Delay1/1
  SignalGen/5(Ramp) -> AmpG/2(Ramp)
  Unit Delay1/1 -> DelayCmp/1(Signal), Product2/1
  SignalGen/2(Amp) -> Product3/1
  Product3/1 -> AmpG/1(Amp)
  DelayCmp/1(UnChange) -> Product2/2, Product3/2
  Product2/1 -> Timer/Enable
  Unit Delay4/1 -> DelayCmp/2(frq)

== system EulerPIDTunning/Controller/PID Controller/Source Model/source: Single ==
  Enable : EnablePort  StatesWhenEnabling=reset
  Add : Sum
  Gain1 : Gain  Gain=Ts
  Sine Wave : Sin  TimeSource=Use external signal  Frequency=Frq*2*pi  SampleTime=31.25e-6
  SineGain : Gain  Gain=VelGain
  Ts : Constant  SampleTime=Ts
  Unit Delay : UnitDelay  SampleTime=Ts
  Sine : Outport  OutputWhenDisabled=reset  InitialOutput=0
  wires:
  Sine Wave/1 -> SineGain/1
  SineGain/1 -> Sine/1
  Add/1 -> Unit Delay/1, Gain1/1
  Ts/1 -> Add/2
  Unit Delay/1 -> Add/1
  Gain1/1 -> Sine Wave/1

== system EulerPIDTunning/Controller/PID Controller/Source Model/source: SineSwp/AmpG ==
  Amp : Inport
  Ramp : Inport  Port=2
  Abs : Abs
  Add1 : Sum  Inputs=+-
  Add2 : Sum
  Product : Product  RndMeth=Zero
  Relational Operator : RelationalOperator  Operator=<=  OutDataTypeStr=boolean  SampleTime=Ts
  Sign : Signum
  Switch : Switch  Threshold=0.5
  Unit Delay1 : UnitDelay  SampleTime=Ts
  TrueAmp : Outport  InitialOutput=0
  wires:
  Add1/1 -> Abs/1, Sign/1
  Add2/1 -> Unit Delay1/1, TrueAmp/1
  Amp/1 -> Add1/1
  Unit Delay1/1 -> Add2/2, Add1/2
  Ramp/1 -> Relational Operator/1, Switch/1
  Abs/1 -> Relational Operator/2, Switch/3
  Relational Operator/1 -> Switch/2
  Switch/1 -> Product/1
  Sign/1 -> Product/2
  Product/1 -> Add2/1

== system EulerPIDTunning/Controller/PID Controller/Source Model/source: SineSwp/DelayCmp ==
  Signal : Inport
  frq : Inport  Port=2
  DelayCmp : Stateflow chart  TreatAsAtomicUnit=on
  Detect Change : simulink/Logic and Bit Operations/Detect Change  SystemSampleTime=-1  vinit=1
  UnChange : Outport
  wires:
  Signal/1 -> Detect Change/1
  Detect Change/1 -> DelayCmp/1(change)
  DelayCmp/1(output) -> UnChange/1
  frq/1 -> DelayCmp/2(frq)

== system EulerPIDTunning/Controller/PID Controller/Source Model/source: SineSwp/Timer ==
  Enable : EnablePort  StatesWhenEnabling=reset
  Add2 : Sum
  Ts : Constant  Value=Ts  SampleTime=Ts
  Unit Delay1 : UnitDelay  SampleTime=Ts
  Time : Outport  OutputWhenDisabled=reset  InitialOutput=0
  wires:
  Ts/1 -> Add2/2
  Unit Delay1/1 -> Add2/1
  Add2/1 -> Time/1, Unit Delay1/1

== matlab function Trajectory Generator/Still/Inverse Kinematic ==
  data: EndPos input double; init_Rot parameter double; Theta output double; L parameter double
function Theta = fcn(EndPos,init_Rot,L)
%#eml
Theta =[0;0; 0; 0; 0; 0];
gd = [init_Rot,EndPos;[0 0 0],1];
[Theta_total,num_total] = inv_kin(gd,L);
%%%%%%%%%%%Need to modify%%%%%%%%%%%%%%%
Theta = Theta_total(:,2);

== matlab function Trajectory Generator/Still/Jacobian ==
  data: Theta input double; Omega output double; EndVel input double; L parameter double
function Omega = fcn(Theta,EndVel,L)
%#eml

Omega = zeros(6,1);
V = [EndVel; 0; 0; 0];   
g = fwd_kin(L,Theta');
Jb = body_Jacobian(L,Theta');
Adg_inv = double(AdjointInv(g));
Omega = double((Jb \ Adg_inv* V)')';

== stateflow chart Controller/PID Controller/Source Model/source: SineSwp/DelayCmp/DelayCmp ==
  state ChechChange
    en:
    output =1 ;
    counter = 0;
  state DealChange
    en:
    output =0 ;
    counter = counter+1;
    du:
    counter = counter+1;
  (default) -> ChechChange
  ChechChange -> DealChange : [change == 1]
  DealChange -> ChechChange : [counter >= 20/frq/Ts]
  data: change input double; output output double; counter local double; frq input double; Ts parameter double

== matlab function Controller/PID Controller/Source Model/source: SineSwp/SignalGen ==
  data: Frq output double; Amp output double; mytime input double; PeriodFlag output double; TureAmp input double; CounterOut output double; CounterIn input double; Ramp output double
function [Frq,Amp,PeriodFlag,CounterOut,Ramp]  = SineGen(mytime,TureAmp, CounterIn)
% This block supports an embeddable subset of the MATLAB language.
% See the help menu for details. 
Ts = 1/8e3;
ii=CounterIn;
% FrqSeries=[10:10:90 100:50:1950 2000:100:5000];
lowfrq = logspace(1,2,50);
medfrq = logspace(2,3,50);
highfrq = logspace(3,log10(2000),20);
% FrqSeries=[lowfrq,medfrq(2:end),highfrq(2:end)];
%  FrqSeries=[medfrq highfrq(2:end)];
%  FrqSeries=lowfrq(10:50);
FrqSeries=highfrq;

% AmpSeries = [0.8 2.5 5 5 repmat(5,[1 74])];
FrqLength=max(size(FrqSeries));
AmpSeries = repmat(5,size(FrqSeries));
% AmpSeries = [repmat(0.8,size(lowfrq)),repmat(5,size(medfrq(2:end))),repmat(5,size(highfrq(2:end)))];

sloptime = 4 ; %period
% PeriodSeries=[repmat(20,size(lowfrq)),repmat(20,size(medfrq(2:end))),repmat(20,size(highfrq(2:end)))]+sloptime; % add 2 acc or dec period;
PeriodSeries=repmat(20,size(FrqSeries))+sloptime;
PeriodTime=PeriodSeries./FrqSeries;

PeriodFlag = 1;             % chech whether the periodn of one frequence finish 
Frq = FrqSeries(ii);
Amp = AmpSeries(ii);
Ramp = Amp*Frq/sloptime*Ts;   % calculate the ramp of Amp; 

if mytime>= PeriodTime(ii) || ii == FrqLength
    Amp = 0;
    if TureAmp <=0
        ii = ii +1;
        if ii >= FrqLength
            ii = FrqLength;
            Amp  = 0;
        end
        PeriodFlag = 0;
    end
else
    PeriodFlag = 1;
end

CounterOut = ii;

== matlab function Trajectory Generator/Circle in Descartes Space/Inverse Kinematic ==
  data: EndPos input double; init_Rot parameter double; Theta output double; L parameter double
function Theta = fcn(EndPos,init_Rot,L)
%#eml
Theta =[0;0; 0; 0; 0; 0];
gd = [init_Rot,EndPos;[0 0 0],1];
[Theta_total,num_total] = inv_kin(gd,L);
%%%%%%%%%%%Need to modify%%%%%%%%%%%%%%%
Theta = Theta_total(:,2);

== matlab function Trajectory Generator/Circle in Descartes Space/Jacobian ==
  data: Theta input double; Omega output double; EndVel input double; L parameter double
function Omega = fcn(Theta,EndVel,L)
%#eml

Omega = zeros(6,1);
V = [EndVel; 0; 0; 0];   
g = fwd_kin(L,Theta');
Jb = body_Jacobian(L,Theta');
Adg_inv = double(AdjointInv(g));
Omega = double((Jb \ Adg_inv* V)')';

== matlab function Trajectory Generator/Line in Joint Space/Forward ==
  data: Theta input double; EndPos output double; L parameter double
function EndPos = fcn(Theta,L)
%#eml
gd = fwd_kin(L,Theta');
EndPos = gd(1:3,4);

== matlab function Trajectory Generator/Line in Joint Space/Jacobian ==
  data: Theta input double; Omega input double; EndVel output double; L parameter double
function EndVel = fcn(Theta,Omega,L)
%#eml


EndVW = spat_Jacobian(L,Theta')*Omega;
gd = fwd_kin(L,Theta');
EndW = EndVW(4:6,1);
gd_pos = gd(1:3,4);
EndVel=cross(EndW,gd_pos);
